simulink model "Ejercicio_1a"  (R2013a)
settings: Solver=ode45  StartTime=0.0  StopTime=10.0  RelTol=1e-3
settings Model: Creator=LuisFernando  LastModifiedBy=LuisFernando

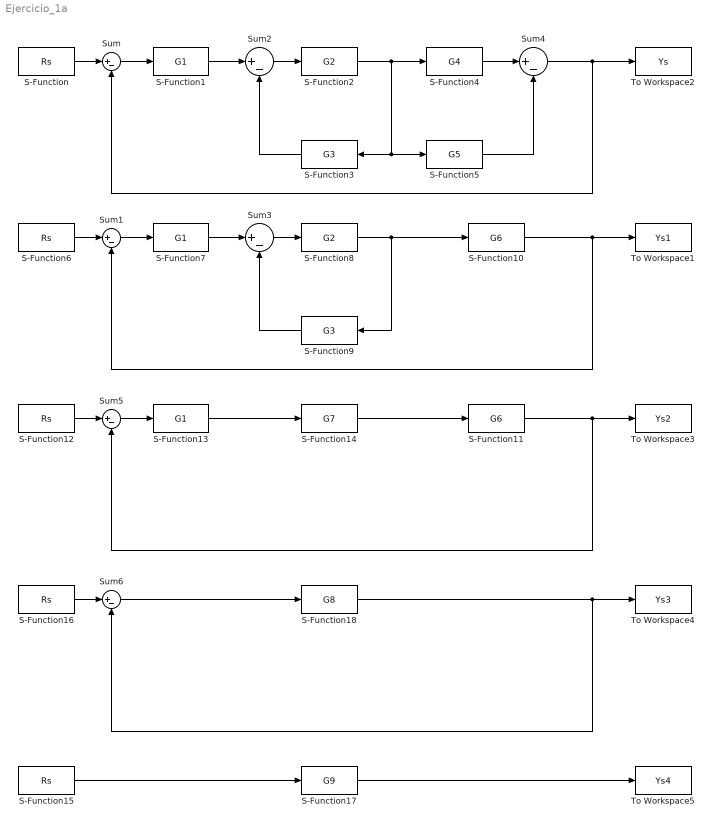
== system Ejercicio_1a ==
  S-Function{,6,12,15..16} (5 alike) : S-Function  FunctionName=Rs  EnableBusSupport=off
  S-Function1 : S-Function  FunctionName=G1  EnableBusSupport=off
  S-Function10 : S-Function  FunctionName=G6  EnableBusSupport=off
  S-Function11 : S-Function  FunctionName=G6  EnableBusSupport=off
  S-Function13 : S-Function  FunctionName=G1  EnableBusSupport=off
  S-Function14 : S-Function  FunctionName=G7  EnableBusSupport=off
  S-Function17 : S-Function  FunctionName=G9  EnableBusSupport=off
  S-Function18 : S-Function  FunctionName=G8  EnableBusSupport=off
  S-Function2 : S-Function  FunctionName=G2  EnableBusSupport=off
  S-Function3 : S-Function  FunctionName=G3  EnableBusSupport=off
  S-Function4 : S-Function  FunctionName=G4  EnableBusSupport=off
  S-Function5 : S-Function  FunctionName=G5  EnableBusSupport=off
  S-Function7 : S-Function  FunctionName=G1  EnableBusSupport=off
  S-Function8 : S-Function  FunctionName=G2  EnableBusSupport=off
  S-Function9 : S-Function  FunctionName=G3  EnableBusSupport=off
  Sum{,1..6} (7 alike) : Sum  Inputs=|+-
  To Workspace1 : ToWorkspace  VariableName=Ys1  SampleTime=-1
  To Workspace2 : ToWorkspace  VariableName=Ys  SampleTime=-1
  To Workspace3 : ToWorkspace  VariableName=Ys2  SampleTime=-1
  To Workspace4 : ToWorkspace  VariableName=Ys3  SampleTime=-1
  To Workspace5 : ToWorkspace  VariableName=Ys4  SampleTime=-1
  wires:
  Sum/1 -> S-Function1/1
  S-Function/1 -> Sum/1
  S-Function1/1 -> Sum2/1
  Sum2/1 -> S-Function2/1
  S-Function3/1 -> Sum2/2
  S-Function2/1 -> S-Function4/1, S-Function5/1, S-Function3/1
  S-Function4/1 -> Sum4/1
  S-Function5/1 -> Sum4/2
  Sum4/1 -> Sum/2, To Workspace2/1
  Sum1/1 -> S-Function7/1
  S-Function6/1 -> Sum1/1
  S-Function7/1 -> Sum3/1
  Sum3/1 -> S-Function8/1
  S-Function9/1 -> Sum3/2
  S-Function8/1 -> S-Function10/1, S-Function9/1
  S-Function10/1 -> Sum1/2, To Workspace1/1
  Sum5/1 -> S-Function13/1
  S-Function12/1 -> Sum5/1
  S-Function13/1 -> S-Function14/1
  S-Function14/1 -> S-Function11/1
  S-Function11/1 -> Sum5/2, To Workspace3/1
  S-Function16/1 -> Sum6/1
  Sum6/1 -> S-Function18/1
  S-Function18/1 -> Sum6/2, To Workspace4/1
  S-Function15/1 -> S-Function17/1
  S-Function17/1 -> To Workspace5/1
